simulink model "RobotX_Click"  (R2024a)
settings: Solver=VariableStepAuto  StartTime=0.0  StopTime=10.0  MaxStep=1e-3  RelTol=1e-3
libraries: simulink x7, aerolibconvert2 x6, RobotX_Lib x2, dspinverses x1, matrix_library x1
settings Model: Creator=margaridaestrela  LastModifiedBy=margaridaestrela

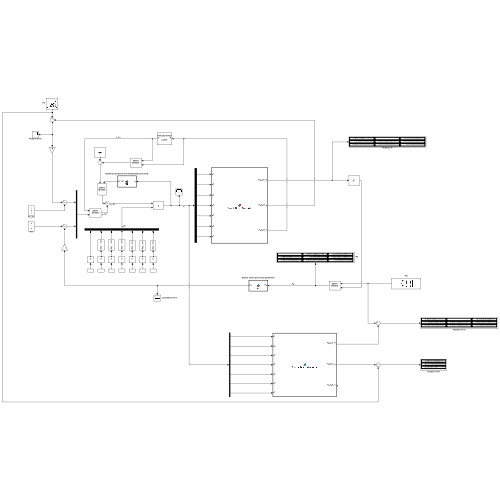
[thumbnail: Simulink's stored preview of the top-level diagram]
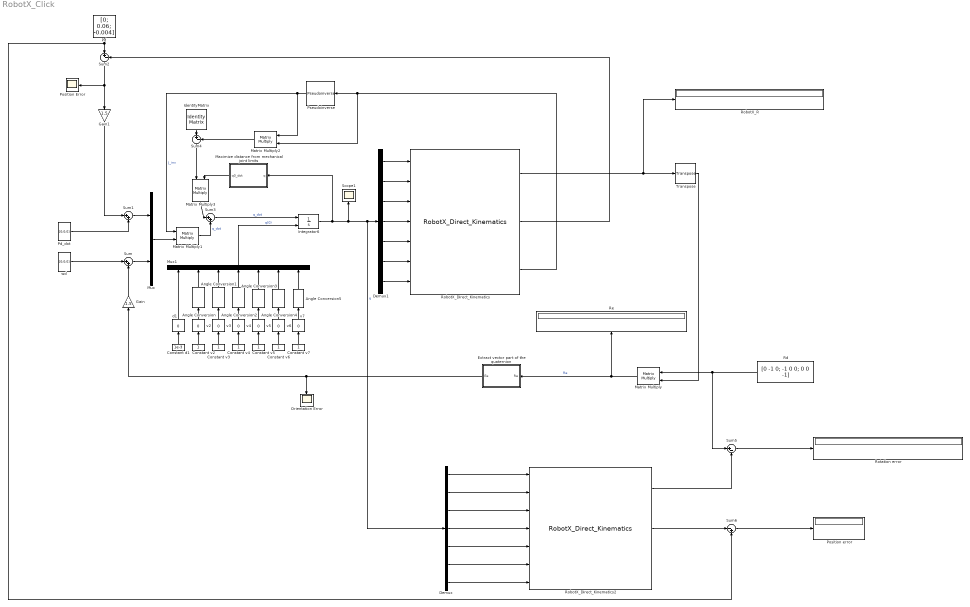
== system RobotX_Click ==
  Angle Conversion{,1..5} (6 alike) : aerolibconvert2/Angle Conversion  IU=deg  OU=rad
  Constant d1 : Constant  Value=1e-3
  Constant v{2..7} (6 alike) : Constant
  Demux : Demux  Outputs=7
  Demux1 : Demux  Outputs=7
  Extract vector part of the quaternion : MATLAB Function  TreatAsAtomicUnit=on
  Gain : Gain  Gain=1.5
  Gain1 : Gain  Gain=1.5
  IdentityMatrix : IdentityMatrix  OutputDimensions=7
  Integrator6 : Integrator  InitialConditionSource=external
  Matrix Multiply{,1..3} (4 alike) : Product  Multiplication=Matrix(*)
  Maximize distance from mechanical joint limits : MATLAB Function  TreatAsAtomicUnit=on
  Mux : Mux  Inputs=2
  Mux1 : Mux  Inputs=7
  Orientation Error : Scope
  Pd : Constant  Value=[0; 0.06; -0.004]  VectorParams1D=off
  Pd_dot : Constant  Value=[0;0;0]  VectorParams1D=off
  Position Error : Scope
  Position error : Display
      settings: Format=decimal (Stored Integer)
  Pseudoinverse : dspinverses/Pseudoinverse  wanterr=off  SimulateUsing=Interpreted execution
  Rd : Constant  Value=[0 -1 0; -1 0 0; 0 0 -1]  VectorParams1D=off
  Re : Display
      settings: Format=decimal (Stored Integer)  Decimation=2
  RobotX_Direct_Kinematics : RobotX_Lib/RobotX_Direct_Kinematics  SystemSampleTime=-1  VariantActivationTime=update diagram  AllowFlexibleInterface=on  Latency=0  AutoFrameSizeCalculation=off
  RobotX_Direct_Kinematics2 : RobotX_Lib/RobotX_Direct_Kinematics  SystemSampleTime=-1  VariantActivationTime=update diagram  AllowFlexibleInterface=on  Latency=0  AutoFrameSizeCalculation=off
  RobotX_R : Display
      settings: Format=decimal (Stored Integer)  Decimation=2
  Rotation error : Display
      settings: Format=decimal (Stored Integer)
  Scope1 : Scope
  Sum : Sum  Inputs=|++
  Sum1 : Sum  Inputs=|++
  Sum2 : Sum  Inputs=|+-
  Sum3 : Sum  Inputs=|++
  Sum4 : Sum  Inputs=|+-
  Sum5 : Sum  Inputs=|+-
  Sum6 : Sum  Inputs=|-+
  Transpose : matrix_library/Transpose
  d1 : simulink/Math Operations/Slider Gain  gain=0  low=-350  high=350
  v2 : simulink/Math Operations/Slider Gain  gain=0  low=-170  high=170
  v3 : simulink/Math Operations/Slider Gain  gain=0  low=-190  high=45
  v4 : simulink/Math Operations/Slider Gain  gain=0  low=-120  high=156
  v5 : simulink/Math Operations/Slider Gain  gain=0  low=-185  high=185
  v6 : simulink/Math Operations/Slider Gain  gain=0  low=-120  high=120
  v7 : simulink/Math Operations/Slider Gain  gain=0  low=-350  high=350
  wd : Constant  Value=[0;0;0]  VectorParams1D=off
  wires:
  Angle Conversion5/1 -> Mux1/7
  Integrator6/1 -> Maximize distance from mechanical joint limits/1(q), Scope1/1, Demux/1, Demux1/1  "q"
  Demux1/1 -> RobotX_Direct_Kinematics/1
  Demux1/2 -> RobotX_Direct_Kinematics/2
  Demux1/3 -> RobotX_Direct_Kinematics/3
  Demux1/4 -> RobotX_Direct_Kinematics/4
  Demux1/5 -> RobotX_Direct_Kinematics/5
  Demux1/6 -> RobotX_Direct_Kinematics/6
  Demux1/7 -> RobotX_Direct_Kinematics/7
  RobotX_Direct_Kinematics/1 -> Transpose/1, RobotX_R/1
  Rd/1 -> Sum5/1, Matrix Multiply/1
  Matrix Multiply/1 -> Extract vector part of the quaternion/1(Re), Re/1  "Re"
  wd/1 -> Sum/1
  Extract vector part of the quaternion/1(Ee) -> Orientation Error/1, Gain/1
  Gain/1 -> Sum/2
  Sum/1 -> Mux/2
  Pd_dot/1 -> Sum1/2
  Gain1/1 -> Sum1/1
  Sum2/1 -> Gain1/1, Position Error/1
  Sum1/1 -> Mux/1
  RobotX_Direct_Kinematics/2 -> Sum2/2
  RobotX_Direct_Kinematics/3 -> Matrix Multiply2/2, Pseudoinverse/1
  Mux/1 -> Matrix Multiply1/2
  Pseudoinverse/1 -> Matrix Multiply1/1, Matrix Multiply2/1  "J_inv"
  Mux1/1 -> Integrator6/2  "q(0)"
  Constant v2/1 -> v2/1
  v5/1 -> Angle Conversion3/1
  v2/1 -> Angle Conversion/1
  Constant d1/1 -> d1/1
  v4/1 -> Angle Conversion2/1
  Constant v5/1 -> v5/1
  Constant v6/1 -> v6/1
  Constant v4/1 -> v4/1
  Constant v3/1 -> v3/1
  v6/1 -> Angle Conversion4/1
  Constant v7/1 -> v7/1
  v7/1 -> Angle Conversion5/1
  v3/1 -> Angle Conversion1/1
  Angle Conversion4/1 -> Mux1/6
  d1/1 -> Mux1/1
  Angle Conversion/1 -> Mux1/2
  Angle Conversion1/1 -> Mux1/3
  Angle Conversion2/1 -> Mux1/4
  Angle Conversion3/1 -> Mux1/5
  IdentityMatrix/1 -> Sum4/1
  Matrix Multiply2/1 -> Sum4/2
  Sum4/1 -> Matrix Multiply3/1
  Sum3/1 -> Integrator6/1  "q_dot"
  Maximize distance from mechanical joint limits/1(q0_dot) -> Matrix Multiply3/2
  Matrix Multiply3/1 -> Sum3/1
  Matrix Multiply1/1 -> Sum3/2  "q_dot"
  Sum5/1 -> Rotation error/1
  Demux/6 -> RobotX_Direct_Kinematics2/6
  Sum6/1 -> Position error/1
  Demux/3 -> RobotX_Direct_Kinematics2/3
  Demux/5 -> RobotX_Direct_Kinematics2/5
  RobotX_Direct_Kinematics2/2 -> Sum6/1
  Demux/7 -> RobotX_Direct_Kinematics2/7
  Demux/1 -> RobotX_Direct_Kinematics2/1
  Demux/4 -> RobotX_Direct_Kinematics2/4
  RobotX_Direct_Kinematics2/1 -> Sum5/2
  Demux/2 -> RobotX_Direct_Kinematics2/2
  Pd/1 -> Sum6/2, Sum2/1
  Transpose/1 -> Matrix Multiply/2

== matlab function RobotX_Click/Maximize distance from mechanical joint limits ==
  data: q0_dot output; q input
function q0_dot = fcn(q)
    n = length(q);
    
    % Manually derive the differentiation
    w_diff = -1 / (2 * n * (pi/2 - (-pi/2)));
    
    q0_dot = 0.01 * w_diff * ones(size(q));
end

== matlab function RobotX_Click/Extract vector part of the quaternion ==
  data: Re input; Ee output
function Ee = fcn(Re)
    Ee = zeros(3, 1);
    trace = Re(1,1) + Re(2,2) + Re(3,3);
    v = acos((trace-1)/2);
    if sin(v) ~= 0
        rx = Re(3, 2) - Re(2, 3);
        ry = Re(1, 3) - Re(3, 1);
        rz = Re(2, 1) - Re(1, 2);

        Ee = 1/(2*sin(v)) * [rx; ry; rz] * v;
    end
end
